simulink subsystem "BackwardAccConverter"  (R2023a)
settings: Solver=VariableStepAuto  StartTime=0.0  StopTime=10.0  RelTol=1e-3
model mask{i_gearbox=0, i_rail=0}
  mask prompts: i_gearbox "ratio of gearbox"; i_rail "ratio of RackAndPinion"
values from neighbouring files (symbols this model uses):
  i_rail = 20 * 1000    (= 20000)    [constants.m]
settings Model: Creator=ПК  LastModifiedBy=ПК

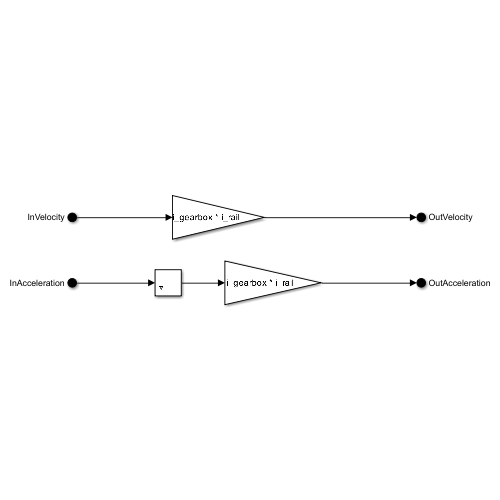
[thumbnail: Simulink's stored preview of the top-level diagram]
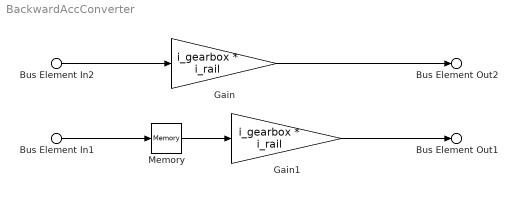
== system BackwardAccConverter ==
  Bus Element In2 : Inport  PortName=InVelocity
  Bus Element In1 : Inport  Port=2  PortName=InAcceleration
  Gain : Gain  Gain=i_gearbox * i_rail
  Gain1 : Gain  Gain=i_gearbox * i_rail
  Memory : Memory
  Bus Element Out2 : Outport  PortName=OutVelocity
  Bus Element Out1 : Outport  Port=2  PortName=OutAcceleration
  wires:
  Bus Element In1/1 -> Memory/1
  Memory/1 -> Gain1/1
  Gain1/1 -> Bus Element Out1/1
  Gain/1 -> Bus Element Out2/1
  Bus Element In2/1 -> Gain/1
